simulink model "Cruise_Control_System"  (R2020a)
settings: Solver=ode45  StartTime=0.0  StopTime=120.0  RelTol=1e-3
values from neighbouring files (symbols this model uses):
  b = 50.0    [CruseControlData.sldd]
  m = 1000.0    [CruseControlData.sldd]
settings Model: DataDictionary=CruseControlData.sldd  Creator=kasutav  LastModifiedBy=kasutav
settings DataIOCC: SaveOutput=off  SaveTime=off

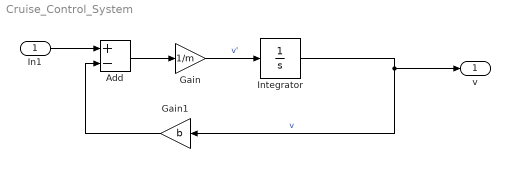
== system Cruise_Control_System ==
  In1 : Inport  OutDataTypeStr=double  PortDimensions=1  SampleTime=0
  Add : Sum  Inputs=+-
  Gain : Gain  Gain=1/m
  Gain1 : Gain  Gain=b
  Integrator : Integrator
  v : Outport  OutDataTypeStr=double  PortDimensions=1  SampleTime=0
  wires:
  In1/1 -> Add/1
  Gain1/1 -> Add/2
  Add/1 -> Gain/1
  Gain/1 -> Integrator/1  "v'"
  Integrator/1 -> Gain1/1, v/1  "v"
